simulink model "emphysema_lung.slx"  (R2023b)
settings: Solver=VariableStepAuto  StartTime=0.0  StopTime=10.0  RelTol=1e-3
settings Model: Creator=R.Dipti  LastModifiedBy=R.Dipti

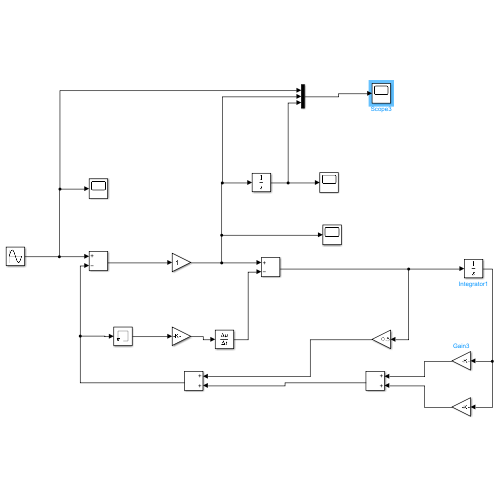
[thumbnail: Simulink's stored preview of the top-level diagram]
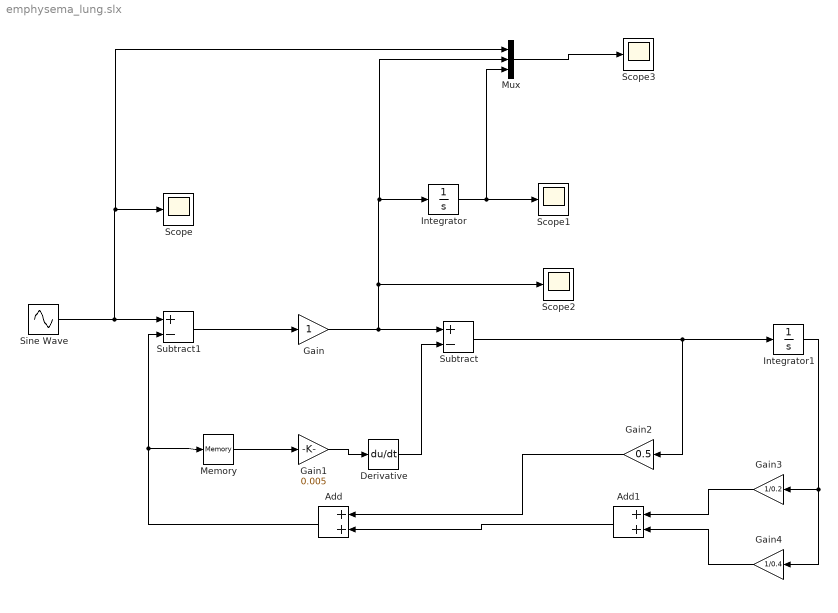
== system emphysema_lung.slx ==
  Add : Sum
  Add1 : Sum
  Derivative : Derivative
  Gain : Gain
  Gain1 : Gain  Gain=0.005
  Gain2 : Gain  Gain=0.5
  Gain3 : Gain  Gain=1/0.2
  Gain4 : Gain  Gain=1/0.4
  Integrator : Integrator
  Integrator1 : Integrator
  Memory : Memory
  Mux : Mux  Inputs=3
  Scope{,1..3} (4 alike) : Scope
  Sine Wave : Sin  SampleTime=0
  Subtract : Sum  Inputs=+-
  Subtract1 : Sum  Inputs=+-
  wires:
  Sine Wave/1 -> Mux/1, Scope/1, Subtract1/1
  Add/1 -> Memory/1, Subtract1/2
  Subtract1/1 -> Gain/1
  Memory/1 -> Gain1/1
  Gain/1 -> Subtract/1, Scope2/1, Mux/2, Integrator/1
  Integrator/1 -> Mux/3, Scope1/1
  Mux/1 -> Scope3/1
  Gain1/1 -> Derivative/1
  Derivative/1 -> Subtract/2
  Subtract/1 -> Gain2/1, Integrator1/1
  Gain2/1 -> Add/1
  Add1/1 -> Add/2
  Gain3/1 -> Add1/1
  Gain4/1 -> Add1/2
  Integrator1/1 -> Gain3/1, Gain4/1
